simulink model "lecture_transfer_functions_model"  (R2018b)
settings: Solver=ode45  StartTime=0.0  StopTime=10.0  RelTol=1e-3  EnableMultiTasking=on
values from neighbouring files (symbols this model uses):
  G_den = [m c k]    [lecture_transfer_functions.m]
  G_num = [1]    [lecture_transfer_functions.m]
  x0 = 1    [lecture_transfer_functions.m]
  xdot0 = -2    [lecture_transfer_functions.m]
settings Model: Creator=lum  LastModifiedBy=Christopher
settings DataIOCC: LimitDataPoints=on  SaveFormat=Array  SignalLoggingSaveFormat=ModelDataLogs
settings OptimizationCC: ExpressionDepthLimit=2147483647  InitFltsAndDblsToZero=on  LifeSpan=inf
settings DebuggingCC: SaveWithParameterizedLinksMsg=none  UnderspecifiedInitializationDetection=Classic  MergeDetectMultiDrivingBlocksExec=none  SolverPrmCheckMsg=warning  FcnCallInpInsideContextMsg=warning  StateNameClashWarn=warning  SFUnexpectedBacktrackingDiag=warning  SFNoUnconditionalDefaultTransitionDiag=warning  SFExecutionAtInitializationDiag=none
settings HardwareCC: ProdBitPerPointer=32  ProdBitPerSizeT=32  ProdBitPerPtrDiffT=32  ProdLargestAtomicFloat=None  ProdIntDivRoundTo=Undefined  ProdEndianess=Unspecified  ProdWordSize=32  ProdHWDeviceType=32-bit Generic
settings ModelReferenceCC: PropagateSignalLabelsOutOfModel=off
settings SFSimCC: SimUseLocalCustomCode=off
settings RTWCC: RTWUseLocalCustomCode=off
settings CodeAppCC: StateflowObjectComments=on
settings GRTTargetCC: TargetFcnLib=ansi_tfl_tmw.mat  TargetLangStandard=C89/C90 (ANSI)  GeneratePreprocessorConditionals=Disable all  CombineOutputUpdateFcns=off  GRTInterface=on
settings ConfigComp: CovMetricSettings=dw  CovHtmlReporting=on  CovSaveCumulativeToWorkspaceVar=on  CovSaveSingleToWorkspaceVar=on  CovExternalEMLEnable=off

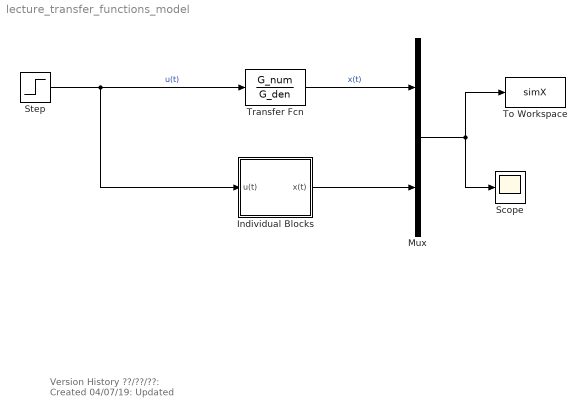
== system lecture_transfer_functions_model ==
  note: Version History
      | ??/??/??: Created
      | 04/07/19: Updated
  Individual Blocks : Subsystem
  Mux : Mux  Inputs=2
  Scope : Scope
  Step : Step  SampleTime=0
  To Workspace : ToWorkspace  VariableName=simX  SaveFormat=Structure With Time  SampleTime=-1
  Transfer Fcn : TransferFcn  Numerator=G_num  Denominator=G_den
  wires:
  Step/1 -> Transfer Fcn/1, Individual Blocks/1(u(t))  "u(t)"
  Transfer Fcn/1 -> Mux/1  "x(t)"
  Individual Blocks/1(x(t)) -> Mux/2
  Mux/1 -> Scope/1, To Workspace/1

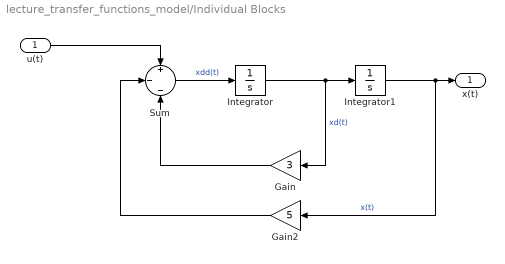
== system lecture_transfer_functions_model/Individual Blocks ==
  u(t) : Inport
  Gain : Gain  Gain=3
  Gain2 : Gain  Gain=5
  Integrator : Integrator  InitialCondition=xdot0
  Integrator1 : Integrator  InitialCondition=x0
  Sum : Sum  Inputs=+|-|-
  x(t) : Outport
  wires:
  Sum/1 -> Integrator/1  "xdd(t)"
  Integrator/1 -> Integrator1/1, Gain/1  "xd(t)"
  Integrator1/1 -> Gain2/1, x(t)/1  "x(t)"
  Gain/1 -> Sum/3
  Gain2/1 -> Sum/2
  u(t)/1 -> Sum/1
